simulink model "MecanumAndObjectDetectionModel"  (R2019b)
settings: Solver=VariableStepAuto  StartTime=0.0  StopTime=inf  RelTol=1e-3
libraries: mobileRoboticsLib x7
settings Model: EnablePacing=on  Creator=spenc  LastModifiedBy=spenc

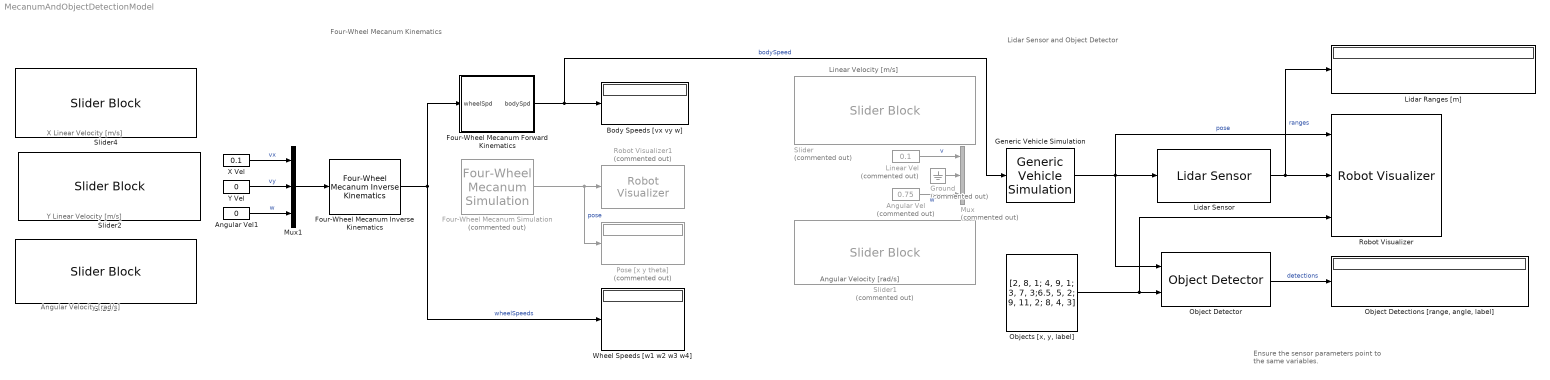
== system MecanumAndObjectDetectionModel ==
  note: Angular Velocity [rad/s]
  note: Lidar Sensor and Object Detector
  note: Ensure the sensor parameters point to the same variables.
  note: Linear Velocity [m/s]
  note: Y Linear Velocity [m/s]
  note: Angular Velocity [rad/s]
  note: X Linear Velocity [m/s]
  note: Four-Wheel Mecanum Kinematics
  Angular Vel : Constant  Commented=on  Value=0.75
  Angular Vel1 : Constant  Value=0
  Body Speeds [vx vy w] : Display
  Four-Wheel Mecanum Forward Kinematics : Subsystem  AncestorBlock=mobileRoboticsLib/Kinematic Models/Four-Wheel Mecanum/Four-Wheel Mecanum Forward Kinematics  mask(Four-Wheel Mecanum Forward Kinematics){wheelRadius=0.1, wheelBase=0.535, wheelTrack=0.459}
      mask prompts: wheelRadius "Wheel Radius [m]"; wheelBase "Wheelbase [m]"; wheelTrack "Track [m]"
      mask help:
      | Calculates the forward kinematics for a four-wheeled vehicle with Mecanum wheels.
      |
      | Input: Wheel speeds [w1; w2; w3; w4] (rad/s)
      |
      | Output: Vehicle velocities [vx; vy; w] in body coordinates (m/s, m/s, and rad/s)
      mask Help: web('matlab:edit mrsDocFourWheelMecanum')
  Four-Wheel Mecanum Inverse Kinematics : mobileRoboticsLib/Kinematic Models/Four-Wheel Mecanum/Four-Wheel Mecanum Inverse Kinematics  wheelRadius=0.1  wheelBase=0.535  wheelTrack=0.459
      settings: SourceProductName=Mobile Robotics Simulation Library
  Four-Wheel Mecanum Simulation : mobileRoboticsLib/Kinematic Models/Four-Wheel Mecanum/Four-Wheel Mecanum Simulation  Commented=on  wheelRadius=0.1  wheelBase=0.535  wheelTrack=0.459  initX=0  initY=0  initAngle=0  Ts=0.05
      settings: SourceProductName=Mobile Robotics Simulation Library
  Generic Vehicle Simulation : mobileRoboticsLib/Utilities/Generic Vehicle Simulation  initX=6  initY=8  initAngle=0  Ts=0.05
      settings: SourceProductName=Mobile Robotics Simulation Library
  Ground : Ground  Commented=on
  Lidar Ranges [m] : Display
  Lidar Sensor : mobileRoboticsLib/Environments/Lidar Sensor  mapName=test_map  sensorOffset=[0,0]  scanAngles=[-pi/4,0,pi/4]  maxRange=5
      settings: SourceProductName=Ground Vehicles Library
  Linear Vel : Constant  Commented=on  Value=0.1
  Mux : Mux  Commented=on  Inputs=3
  Mux1 : Mux  Inputs=3
  "Object Detections [range, angle, label]" : Display
  Object Detector : mobileRoboticsLib/Environments/Object Detector  mapName=test_map  sensorOffset=[0,0]  sensorAngle=0  fieldOfView=pi/3  maxRange=5  maxDetections=3  sampleTime=0.1
      settings: SourceProductName=Ground Vehicles Library
  "Objects [x, y, label]" : Constant  Value=[2, 8, 1; 4, 9, 1; 3, 7, 3;6.5, 5, 2; 9, 11, 2; 8, 4, 3]
  Pose [x y theta] : Display  Commented=on
  Robot Visualizer : mobileRoboticsLib/Environments/Robot Visualizer  Priority=99  robotRadius=0.5  mapName=test_map  showTrajectory=off  hasWaypoints=off  hasLidar=on  sensorOffset=[0,0]  scanAngles=[-pi/4,0,pi/4]  hasObjDetector=on  objDetectorOffset=[0,0]  objDetectorAngle=0  objDetectorFOV=pi/4  objDetectorMaxRange=5  objectColors=eye(3,3)  objectMarkers=s
      settings: SourceProductName=Ground Vehicles Library
  Robot Visualizer1 : mobileRoboticsLib/Environments/Robot Visualizer  Priority=99  Commented=on  robotRadius=0  showTrajectory=on  hasWaypoints=off  hasLidar=off  sensorOffset=[ 0 0 ]  scanAngles=scanAngles  hasObjDetector=off  objDetectorOffset=[ 0, 0 ]  objDetectorAngle=0  objDetectorFOV=pi/4  objDetectorMaxRange=5  objectColors=[ 1, 0, 0; 0, 1, 0; 0, 0, 1 ]  objectMarkers=s
      settings: SourceProductName=Ground Vehicles Library
  Slider : SliderBlock  Commented=on  ScaleMax=1
  Slider1 : SliderBlock  Commented=on  ScaleMin=-1.5  ScaleMax=1.5
  Slider2 : SliderBlock  ScaleMin=-1  ScaleMax=1  TickInterval=0.25
  Slider3 : SliderBlock  ScaleMin=-1.5  ScaleMax=1.5
  Slider4 : SliderBlock  ScaleMin=-1  ScaleMax=1  TickInterval=0.25
  Wheel Speeds [w1 w2 w3 w4] : Display
  X Vel : Constant  Value=0.1
  Y Vel : Constant  Value=0
  wires:
  Lidar Sensor/1 -> Lidar Ranges [m]/1, Robot Visualizer/2  "ranges"
  Ground/1 -> Mux/2
  "Objects [x, y, label]"/1 -> Robot Visualizer/3, Object Detector/2
  Object Detector/1 -> "Object Detections [range, angle, label]"/1  "detections"
  Generic Vehicle Simulation/1 -> Lidar Sensor/1, Robot Visualizer/1, Object Detector/1  "pose"
  Linear Vel/1 -> Mux/1  "v"
  Angular Vel/1 -> Mux/3  "w"
  Four-Wheel Mecanum Inverse Kinematics/1 -> Four-Wheel Mecanum Forward Kinematics/1(wheelSpd), Wheel Speeds [w1 w2 w3 w4]/1  "wheelSpeeds"
  X Vel/1 -> Mux1/1  "vx"
  Four-Wheel Mecanum Simulation/1 -> Pose [x y theta]/1, Robot Visualizer1/1  "pose"
  Mux1/1 -> Four-Wheel Mecanum Inverse Kinematics/1
  Y Vel/1 -> Mux1/2  "vy"
  Angular Vel1/1 -> Mux1/3  "w"
  Four-Wheel Mecanum Forward Kinematics/1(bodySpd) -> Generic Vehicle Simulation/1, Body Speeds [vx vy w]/1  "bodySpeed"

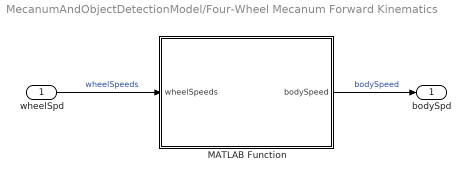
== system MecanumAndObjectDetectionModel/Four-Wheel Mecanum Forward Kinematics ==
  wheelSpd : Inport
  MATLAB Function : MATLAB Function  TreatAsAtomicUnit=on
  bodySpd : Outport  VectorParamsAs1DForOutWhenUnconnected=off
  wires:
  wheelSpd/1 -> MATLAB Function/1(wheelSpeeds)  "wheelSpeeds"
  MATLAB Function/1(bodySpeed) -> bodySpd/1  "bodySpeed"

== matlab function MecanumAndObjectDetectionModel/Four-Wheel Mecanum Forward Kinematics/MATLAB Function ==
  settings: updateMethod=DISCRETE
  data: wheelSpeeds input; bodySpeed output; wheelRadius parameter; wheelBase parameter; wheelTrack parameter
function bodySpeed = fourWheelMecanumFwdKin(wheelSpeeds,wheelRadius,wheelBase,wheelTrack)
    
    % Initialize FourWheelMecanum object
%% 
    persistent robot
    if isempty(robot)
        robot = FourWheelMecanum(wheelRadius,wheelBase,wheelTrack);
    end
    
    % Run object's forward kinematics method
    bodySpeed = forwardKinematics(robot,wheelSpeeds);

end
